simulink model "aeropendulum_dynamics"  (R2023b)
settings: Solver=FixedStepAuto  StartTime=0.0  StopTime=10  FixedStep=0.0001  RelTol=1e-3
libraries: slpidlib x1
settings Model: Creator=davi_  LastModifiedBy=davi_

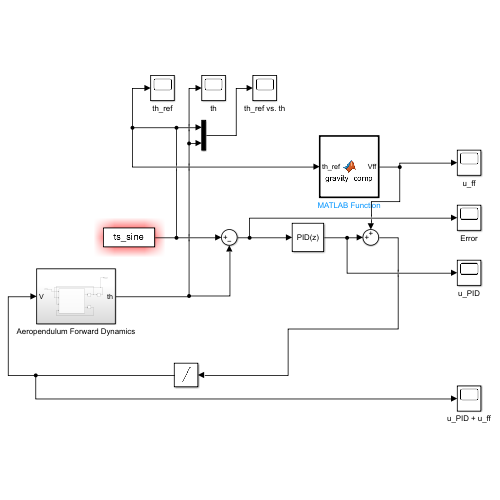
[thumbnail: Simulink's stored preview of the top-level diagram]
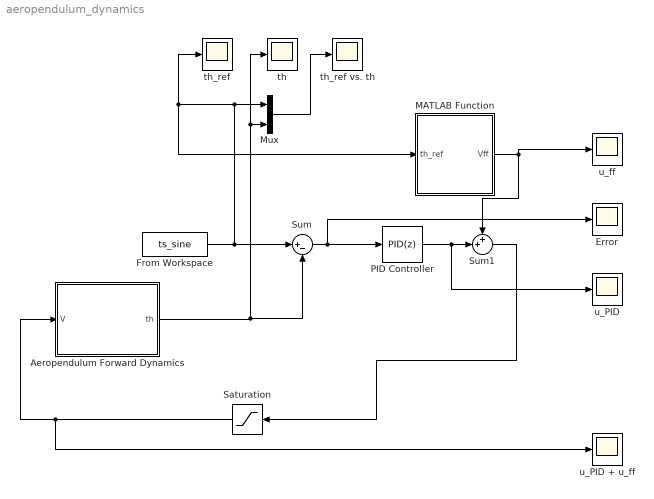
== system aeropendulum_dynamics ==
  Aeropendulum Forward Dynamics : Subsystem
  Error : Scope
  From Workspace : FromWorkspace  VariableName=ts_sine
  MATLAB Function : MATLAB Function  TreatAsAtomicUnit=on
  Mux : Mux  Inputs=2
  PID Controller : slpidlib/PID Controller  Controller=PID  Form=Parallel  TimeDomain=Discrete-time  UseExternalTs=off  SampleTime=0.001  IntegratorMethod=Forward Euler  FilterMethod=Forward Euler  ControllerParametersSource=internal  P=2.5  I=1.5  UseKiTs=off  D=1  N=50  UseFilter=on  TunerSelectOption=Transfer Function Based (PID Tuner App)  InitialConditionSource=internal  InitialConditionForIntegrator=0  InitialConditionForFilter=0  DifferentiatorICPrevScaledInput=0  ExternalReset=none  TrackingMode=off  Kt=1  LimitOutput=off  SatLimitsSource=internal  UpperSaturationLimit=inf  LowerSaturationLimit=-inf  LinearizeAsGain=on  AntiWindupMode=none  Kb=1  LimitIntegrator=off  UpperIntegratorSaturationLimit=inf  LowerIntegratorSaturationLimit=-inf  POutMin=[]  POutMax=[]  IOutMin=[]  IOutMax=[]  DOutMin=[]  DOutMax=[]  NOutMin=[]  NOutMax=[]  SumOutMin=[]  SumOutMax=[]  SaturationOutMin=[]  SaturationOutMax=[]  PParamMin=[]  PParamMax=[]  IParamMin=[]  IParamMax=[]  DParamMin=[]  DParamMax=[]  NParamMin=[]  NParamMax=[]  KbParamMin=[]  KbParamMax=[]  KtParamMin=[]  KtParamMax=[]  KbOutMin=[]  KbOutMax=[]  KtOutMin=[]  KtOutMax=[]  IntegratorOutMin=[]  IntegratorOutMax=[]  FilterOutMin=[]  FilterOutMax=[]  SumI1OutMin=[]  SumI1OutMax=[]  SumI2OutMin=[]  SumI2OutMax=[]  SumI3OutMin=[]  SumI3OutMax=[]  SumI4OutMin=[]  SumI4OutMax=[]  SumDOutMin=[]  SumDOutMax=[]  DifferentiatorOutMin=[]  DifferentiatorOutMax=[]  FilterDiffOutCoefMin=[]  FilterDiffOutCoefMax=[]  ReciprocalOutMin=[]  ReciprocalOutMax=[]  SumDenOutMin=[]  SumDenOutMax=[]  SumNumOutMin=[]  SumNumOutMax=[]  DivideOutMin=[]  DivideOutMax=[]  UdiffTsProdOutMin=[]  UdiffTsProdOutMax=[]  NTsProdOutMin=[]  NTsProdOutMax=[]  UintegralTsProdOutMin=[]  UintegralTsProdOutMax=[]  UngainTsProdOutMin=[]  UngainTsProdOutMax=[]  ClampingZeroOutDataTypeStr=Inherit: Inherit via back propagation  ClampingZeroOutMin=[]  ClampingZeroOutMax=[]  FilterDenConstantOutDataTypeStr=Inherit: Inherit via back propagation  FilterDenConstantOutMin=[]  FilterDenConstantOutMax=[]  PCopyOutDataTypeStr=Inherit: Inherit via back propagation  PCopyOutMin=[]  PCopyOutMax=[]  NCopyOutDataTypeStr=Inherit: Inherit via back propagation  NCopyOutMin=[]  NCopyOutMax=[]  IntegratorContinuousStateAttributes=''  IntegratorStateMustResolveToSignalObject=off  IntegratorRTWStateStorageClass=Auto  FilterContinuousStateAttributes=''  FilterStateMustResolveToSignalObject=off  FilterRTWStateStorageClass=Auto  ParallelPVariant=InternalParameters  IdealPVariant=Disabled  IVariant=InternalParameters  DVariant=InternalParameters  IntegratorVariant=Discrete  SatVariant=Disabled  AWVariant=Passthrough  PCopyVariant=Disabled  TRVariant=Disabled  FdbkBlocksVariant=Forward  IdealPFdbkVariant=Disabled  SatFdbkVariant=Disabled  DerivativeFilterVariant=ForwardEulerFilter  NVariant=InternalParameters  NCopyVariant=Disabled  FilterICVariant=InternalICsFilter  IntegratorICVariant=InternalICs  ExternalResetVariant=Disabled  TRSumVariant=Passthrough  SumFdbkVariant=Disabled  SumVariant=Sum_PID  TsampFilterVariant=InternalTs  TsampNgainVariant=Passthrough  TsampIntegralVariant=Disabled_SignalSpec  ExternalSaturationOutDataTypeStr=Inherit: Same as second input
  Saturation : Saturate  UpperLimit=12  LowerLimit=0
  Sum : Sum  Inputs=|+-
  Sum1 : Sum  Inputs=++|
  th : Scope
  th_ref : Scope
  th_ref vs. th : Scope
  u_PID : Scope
  u_PID + u_ff : Scope
  u_ff : Scope
  wires:
  Aeropendulum Forward Dynamics/1(th) -> Sum/2, Mux/2, th/1
  Sum/1 -> PID Controller/1, Error/1
  PID Controller/1 -> u_PID/1, Sum1/2
  Saturation/1 -> u_PID + u_ff/1, Aeropendulum Forward Dynamics/1(V)
  From Workspace/1 -> th_ref/1, MATLAB Function/1(th_ref), Mux/1, Sum/1
  Mux/1 -> th_ref vs. th/1
  MATLAB Function/1(Vff) -> u_ff/1, Sum1/1
  Sum1/1 -> Saturation/1

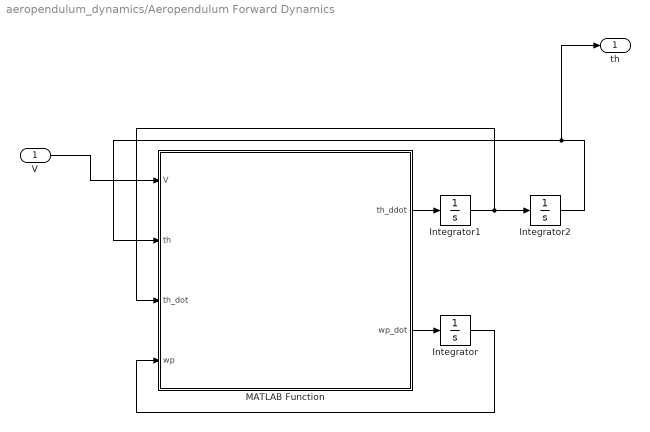
== system aeropendulum_dynamics/Aeropendulum Forward Dynamics ==
  V : Inport
  Integrator : Integrator
  Integrator1 : Integrator
  Integrator2 : Integrator
  MATLAB Function : MATLAB Function  TreatAsAtomicUnit=on
  th : Outport
  wires:
  MATLAB Function/1(th_ddot) -> Integrator1/1
  Integrator1/1 -> Integrator2/1, MATLAB Function/3(th_dot)
  Integrator/1 -> MATLAB Function/4(wp)
  Integrator2/1 -> th/1, MATLAB Function/2(th)
  MATLAB Function/2(wp_dot) -> Integrator/1
  V/1 -> MATLAB Function/1(V)

== matlab function aeropendulum_dynamics/MATLAB Function ==
  data: Vff output; th_ref input; p parameter
function Vff = gravity_comp(th_ref, p)

% GRAVITY_COMP Calculates the feedforward gravity compensation control
% action through calculating the actuator's inverse dynamics


% 1. Actuator Inverse Dynamics (Vff)
    Vff = (1/p.K_v)*sqrt((p.m_p*p.L_cm_p + p.m_l*p.r)*p.g*cos(th_ref)/(p.L_p*p.k_T));

== matlab function aeropendulum_dynamics/Aeropendulum Forward Dynamics/MATLAB Function ==
  data: V input; th_ddot output; th input; th_dot input; wp input; wp_dot output; p parameter
function [th_ddot, wp_dot] = aeropendulum_dynamics(V, th, th_dot, wp, p)
% AEROPENDULUM_DYNAMICS Calculates the forward dynamics of the system.
%
% This block receives the physical parameters via the struct 'p' to ensure 
% a Single Source of Truth and avoid base workspace pollution.

    % 1. Actuator Dynamics (w_p_dot)
    wp_dot = (1 / p.tau_m) * (p.K_v * V - wp);
    
    % 2. Mechanical Dynamics (theta_ddot)
    v_prop = th_dot * p.L_p;
    F_t = (p.k_T * wp^2) - (p.k_adv * v_prop * wp);
    tau_t = F_t * p.L_p; % Thrust torque
    
    tau_ad = p.C_d * th_dot * abs(th_dot); % Aerodynamic drag torque
    tau_g = p.m * p.g * p.L_cm * cos(th);  % Gravity torque (th=0 is horizontal)
    tau_f = p.B_eq * th_dot;               % Friction torque
    tau_l = 0;                             % External load torque
    
    % Angular acceleration
    th_ddot = (1 / p.J) * (tau_t - tau_g - tau_f - tau_ad - tau_l);
end
